simulink model "SD2_DEM"  (Simulink 6.0)
settings: Solver=ode45  StartTime=0.0  StopTime=100*Ts  RelTol=1e-3
undefined symbols (not defined in the file or in its folder): Ampl, DEM, DEM_sel, Fin, flag_dac, flag_quant, Fs, LSB, mism, Nelements, offset, quantizer, Ts, VfsH, VfsL, vth, vthid
settings Model: Creator=ivan  LastModifiedBy=Cri  ExtModeAutoUpdateStatusClock=off

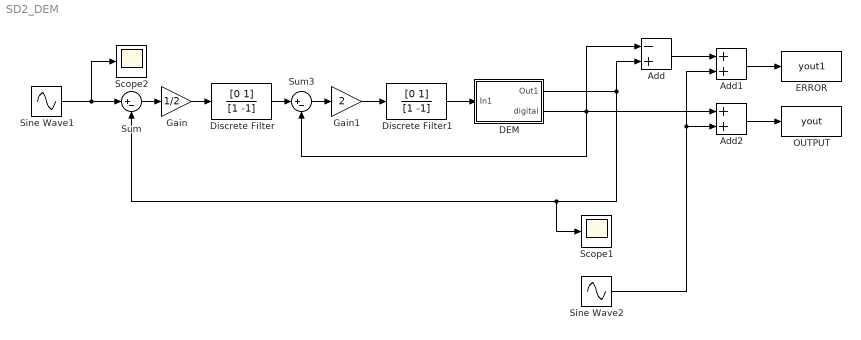
== system SD2_DEM ==
  Add : Sum  Inputs=-+  OutScaling=2^-10
  Add1 : Sum  OutScaling=2^-10
  Add2 : Sum  OutScaling=2^-10
  DEM : Subsystem
      mask Display:
      | color('black');disp('DEM')
      | port_label('output', 2, 'dig')
      | port_label('output', 1, 'an')
      | port_label('input', 1, 'in')
  Discrete Filter : DiscreteFilter  Numerator=[0 1]  Denominator=[1 -1]  SampleTime=Ts
  Discrete Filter1 : DiscreteFilter  Numerator=[0 1]  Denominator=[1 -1]  SampleTime=Ts
  ERROR : ToWorkspace  VariableName=yout1  SampleTime=Ts  SaveFormat=Array
  Gain : Gain  Gain=1/2
  Gain1 : Gain  Gain=2
  OUTPUT : ToWorkspace  VariableName=yout  SampleTime=Ts  SaveFormat=Array
  Scope1 : Scope
      settings: TimeRange=1.440997229916899e-006  YMin=-0.705989  YMax=0.466618
  Scope2 : Scope
      settings: TimeRange=1.440997229916899e-006  YMin=-0.705989  YMax=0.466618
  Sine Wave1 : Sin  Amplitude=Ampl  Bias=offset  Frequency=2*pi*Fin  SampleTime=Ts
  Sine Wave2 : Sin  Amplitude=(VfsH - VfsL)/2  Bias=offset  Frequency=2*pi*Fs/2  Phase=pi/4  SampleTime=Ts
  Sum : Sum  Inputs=|+-
  Sum3 : Sum  Inputs=|+-
  wires:
  Sine Wave1/1 -> Sum/1, Scope2/1
  Sum/1 -> Gain/1
  Discrete Filter/1 -> Sum3/1
  Sum3/1 -> Gain1/1
  Gain/1 -> Discrete Filter/1
  Gain1/1 -> Discrete Filter1/1
  DEM/1(Out1) -> Scope1/1, Sum/2, Add/2
  DEM/2(digital) -> Sum3/2, Add2/1, Add/1
  Discrete Filter1/1 -> DEM/1(In1)
  Add1/1 -> ERROR/1
  Add/1 -> Add1/1
  Sine Wave2/1 -> Add1/2, Add2/2
  Add2/1 -> OUTPUT/1

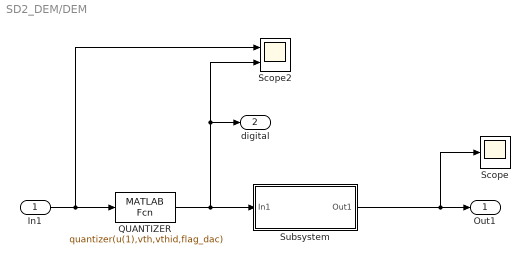
== system SD2_DEM/DEM ==
  In1 : Inport  Port=1  LatchInput=off
  QUANTIZER : MATLABFcn  MATLABFcn=quantizer(u(1),vth,vthid,flag_dac)  OutputDimensions=1  OutputSignalType=real  SampleTime=Ts
  Scope : Scope
      settings: SaveName=ScopeData2
  Scope2 : Scope  NumInputPorts=2
      settings: YMin=0.62035~-5  YMax=0.68565~5  SaveName=ScopeData5
  Subsystem : Subsystem
      mask Display: disp('DEM')
  Out1 : Outport
  digital : Outport  Port=2
  wires:
  QUANTIZER/1 -> Subsystem/1(In1), digital/1, Scope2/2
  In1/1 -> QUANTIZER/1, Scope2/1
  Subsystem/1(Out1) -> Out1/1, Scope/1

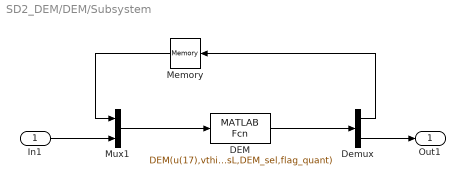
== system SD2_DEM/DEM/Subsystem ==
  In1 : Inport  Port=1  LatchInput=off
  DEM : MATLABFcn  MATLABFcn=DEM(u(17),vthid,flag_dac,mism,u(1),u(2),u(3),u(4),u(5),u(6),u(7),u(8),u(9),u(10),u(11),u(12),u(13),u(14),u(15),u(16),Nelements,LSB,VfsL,DEM_sel,flag_quant)  OutputDimensions=17  OutputSignalType=real  Output1D=off  SampleTime=Ts
  Demux : Demux  Outputs=2
  Memory : Memory  Orientation=left  X0=1  InheritSampleTime=on  LinearizeMemory=on
  Mux1 : Mux  Inputs=2
  Out1 : Outport
  wires:
  Mux1/1 -> DEM/1
  In1/1 -> Mux1/2
  DEM/1 -> Demux/1
  Demux/1 -> Memory/1
  Demux/2 -> Out1/1
  Memory/1 -> Mux1/1
